simulink model "assignment2_PI"  (R2016a)
settings: Solver=VariableStepAuto  StartTime=0.0  StopTime=2000  RelTol=1e-3
values from neighbouring files (symbols this model uses):
  A = [ -0.005131 0 0 0 0 ... (first row only)    [assgt2.m]
  B = [ -0.629 0.624 ... (first row only)    [assgt2.m]
  Bd = [ -0.062 -0.067 ... (first row only)    [assgt2.m]
  C = [ -0.7223 -0.5170 0.3386 -0.1633 0.1121 ... (first row only)    [assgt2.m]
  Ki = [1/Ti1 0 ... (first row only)    [assgt2.m]
  Kp = [0.2 0 ... (first row only)    [assgt2.m]
settings Model: Creator=Sondre  LastModifiedBy=Sondre

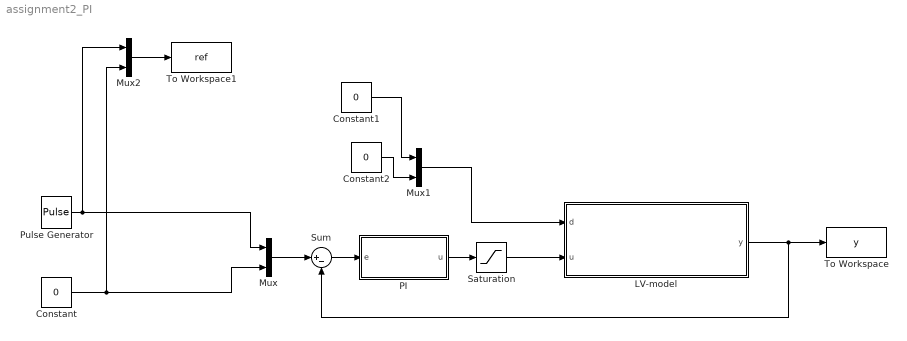
== system assignment2_PI ==
  Constant : Constant  Value=0
  Constant1 : Constant  Value=0
  Constant2 : Constant  Value=0
  LV-model : Subsystem
  Mux : Mux  Inputs=2
  Mux1 : Mux  Inputs=2
  Mux2 : Mux  Inputs=2
  "PI " : Subsystem
  Pulse Generator : DiscretePulseGenerator  PulseType=Time based  Period=200  PulseWidth=50  PhaseDelay=100
  Saturation : Saturate
  Sum : Sum  Inputs=|+-
  To Workspace : ToWorkspace  VariableName=y  SaveFormat=Timeseries  SampleTime=-1
  To Workspace1 : ToWorkspace  VariableName=ref  SaveFormat=Timeseries  SampleTime=-1
  wires:
  LV-model/1(y) -> Sum/2, To Workspace/1
  "PI "/1("u ") -> Saturation/1
  Sum/1 -> "PI "/1("e ")
  Mux/1 -> Sum/1
  Constant/1 -> Mux2/2, Mux/2
  Pulse Generator/1 -> Mux2/1, Mux/1
  Constant1/1 -> Mux1/1
  Constant2/1 -> Mux1/2
  Mux1/1 -> LV-model/1(d)
  Mux2/1 -> To Workspace1/1
  Saturation/1 -> LV-model/2(u)

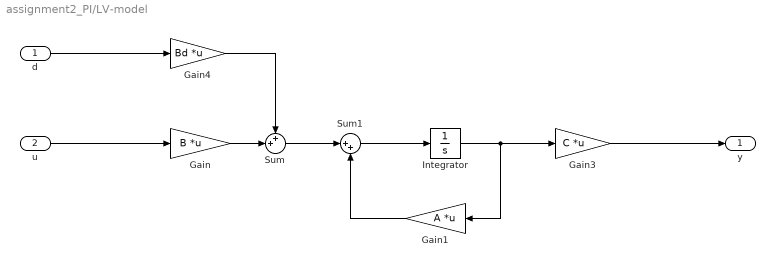
== system assignment2_PI/LV-model ==
  d : Inport
  u : Inport  Port=2
  Gain : Gain  Gain=B  Multiplication=Matrix(K*u)
  Gain1 : Gain  Gain=A  Multiplication=Matrix(K*u)
  Gain3 : Gain  Gain=C  Multiplication=Matrix(K*u)
  Gain4 : Gain  Gain=Bd  Multiplication=Matrix(K*u)
  Integrator : Integrator
  Sum : Sum  Inputs=++|
  Sum1 : Sum  Inputs=|++
  y : Outport
  wires:
  d/1 -> Gain4/1
  Gain4/1 -> Sum/1
  Gain1/1 -> Sum1/2
  Gain/1 -> Sum/2
  Sum/1 -> Sum1/1
  Gain3/1 -> y/1
  Sum1/1 -> Integrator/1
  Integrator/1 -> Gain1/1, Gain3/1
  u/1 -> Gain/1

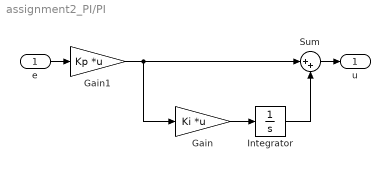
== system assignment2_PI/PI  ==
  "e " : Inport
  Gain : Gain  Gain=Ki  Multiplication=Matrix(K*u)
  Gain1 : Gain  Gain=Kp  Multiplication=Matrix(K*u)
  Integrator : Integrator
  Sum : Sum  Inputs=|++
  "u " : Outport
  wires:
  Sum/1 -> "u "/1
  "e "/1 -> Gain1/1
  Gain/1 -> Integrator/1
  Integrator/1 -> Sum/2
  Gain1/1 -> Gain/1, Sum/1
